simulink model "baicuoiki"  (R2017b)
settings: Solver=FixedStepAuto  StartTime=0.0  StopTime=50  FixedStep=0.01  RelTol=1e-3
settings Model: Creator=ADMIN  LastModifiedBy=ADMIN

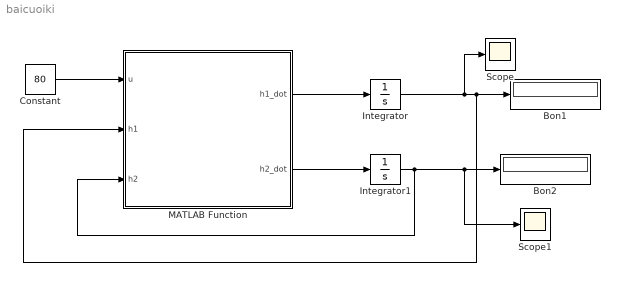
== system baicuoiki ==
  Bon1 : Display
  Bon2 : Display
  Constant : Constant  Value=80
  Integrator : Integrator  InitialCondition=0.01
  Integrator1 : Integrator  InitialCondition=0.01
  MATLAB Function : MATLAB Function  TreatAsAtomicUnit=on
  Scope : Scope
  Scope1 : Scope
  wires:
  Constant/1 -> MATLAB Function/1(u)
  Integrator1/1 -> Scope1/1, Bon2/1, MATLAB Function/3(h2)
  Integrator/1 -> Scope/1, Bon1/1, MATLAB Function/2(h1)
  MATLAB Function/1(h1_dot) -> Integrator/1
  MATLAB Function/2(h2_dot) -> Integrator1/1

== matlab function baicuoiki/MATLAB Function ==
  data: u input; h1_dot output; h1 input; h2 input; h2_dot output
function [h1_dot, h2_dot] = fcn(u,h1,h2)

%#codegen
A1 = 175;      % cm^2
A2 = 154;      % cm^2
b1 = 1.1;      % cm^2
b2 = 1.0;      % cm^2
K = 41;        % cm^3/s/V
C = 0.6;
g = 981;       % cm/s^2
h1_dot=(K*u-sign(h1-h2)*b1*C*sqrt(2*g*abs(h1-h2)))/A1;
h2_dot=(sign(h1-h2)*b1*C*sqrt(2*g*abs(h1-h2))-b2*C*sqrt(2*g*h2))/A2;
